simulink model "Mdl_Actuator"  (R2019b)
settings: Solver=FixedStepAuto  StartTime=0.0  StopTime=10.0  FixedStep=DT  RelTol=1e-3
values from neighbouring files (symbols this model uses):
  kappa = 0.01    [DD_Mdl_Actuator.sldd]
  tau = 0.01    [DD_Mdl_Actuator.sldd]
settings Model: DataDictionary=DD_Mdl_Actuator.sldd  Creator=ditt_aj  LastModifiedBy=ditt_aj

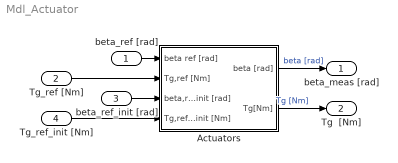
== system Mdl_Actuator ==
  beta_ref [rad] : Inport
  Tg_ref [Nm] : Inport  Port=2
  beta_ref_init [rad] : Inport  Port=3
  Tg_ref_init [Nm] : Inport  Port=4
  Actuators : Subsystem
  "beta_meas [rad] " : Outport  VectorParamsAs1DForOutWhenUnconnected=off
  Tg  [Nm] : Outport  Port=2  VectorParamsAs1DForOutWhenUnconnected=off
  wires:
  beta_ref [rad]/1 -> Actuators/1(beta ref [rad])
  Tg_ref [Nm]/1 -> Actuators/2(Tg,ref [Nm])
  Actuators/2(Tg[Nm]) -> Tg  [Nm]/1  "Tg [Nm]"
  Tg_ref_init [Nm]/1 -> Actuators/4(Tg,ref init [Nm])
  Actuators/1(beta [rad]) -> "beta_meas [rad] "/1  "beta [rad]"
  beta_ref_init [rad]/1 -> Actuators/3(beta,ref init [rad])

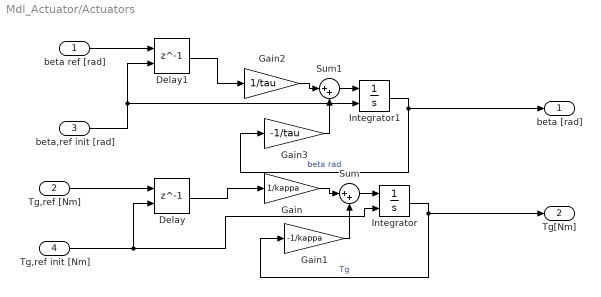
== system Mdl_Actuator/Actuators ==
  beta ref [rad] : Inport
  Tg,ref [Nm] : Inport  Port=2
  beta,ref init [rad] : Inport  Port=3
  Tg,ref init [Nm] : Inport  Port=4
  Delay : Delay  DelayLength=1  InitialConditionSource=Input port
      settings: InputPortMap=u0,p4
  Delay1 : Delay  DelayLength=1  InitialConditionSource=Input port
      settings: InputPortMap=u0,p4
  Gain : Gain  Gain=1/kappa
  Gain1 : Gain  Gain=-1/kappa
  Gain2 : Gain  Gain=1/tau
  Gain3 : Gain  Gain=-1/tau
  Integrator : Integrator  InitialConditionSource=external
  Integrator1 : Integrator  InitialConditionSource=external
  Sum : Sum  Inputs=|++
  Sum1 : Sum  Inputs=|++
  beta [rad] : Outport  VectorParamsAs1DForOutWhenUnconnected=off
  Tg[Nm] : Outport  Port=2  VectorParamsAs1DForOutWhenUnconnected=off
  wires:
  Sum1/1 -> Integrator1/1
  Integrator/1 -> Tg[Nm]/1, Gain1/1  "Tg"
  Tg,ref init [Nm]/1 -> Delay/2, Integrator/2
  Gain3/1 -> Sum1/2
  Gain2/1 -> Sum1/1
  Sum/1 -> Integrator/1
  Gain1/1 -> Sum/2
  Integrator1/1 -> beta [rad]/1, Gain3/1  "beta rad"
  Gain/1 -> Sum/1
  Tg,ref [Nm]/1 -> Delay/1
  Delay/1 -> Gain/1
  beta ref [rad]/1 -> Delay1/1
  Delay1/1 -> Gain2/1
  beta,ref init [rad]/1 -> Integrator1/2, Delay1/2
